simulink model "Step_11"  (R2024b)
settings: Solver=VariableStepAuto  StartTime=0.0  StopTime=100.0  RelTol=1e-3
libraries: simulink x1
settings Model: Creator=Omar

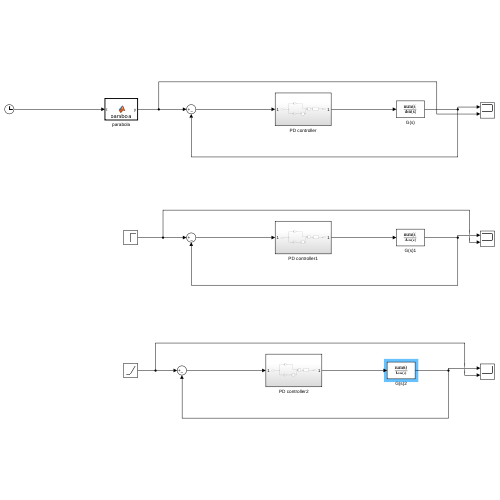
[thumbnail: Simulink's stored preview of the top-level diagram]
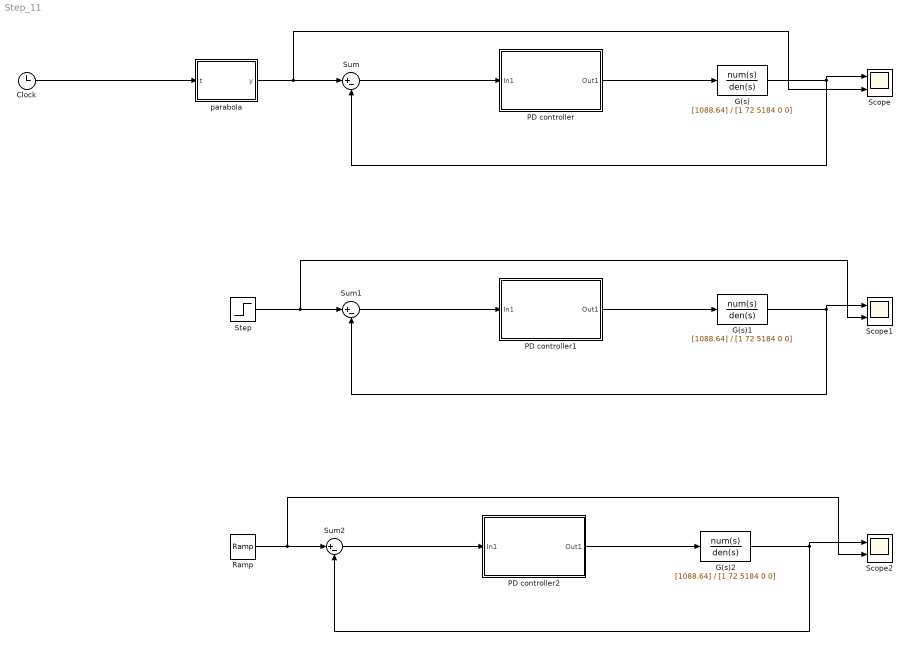
== system Step_11 ==
  Clock : Clock
      settings: Decimation=100
  G(s) : TransferFcn  Numerator=[1088.64]  Denominator=[1 72 5184 0 0]
  G(s)1 : TransferFcn  Numerator=[1088.64]  Denominator=[1 72 5184 0 0]
  G(s)2 : TransferFcn  Numerator=[1088.64]  Denominator=[1 72 5184 0 0]
  PD controller : Subsystem
  PD controller1 : Subsystem
  PD controller2 : Subsystem
  Ramp : simulink/Sources/Ramp  slope=1  start=0  InitialOutput=0
  Scope : Scope  NumInputPorts=2
  Scope1 : Scope  NumInputPorts=2
  Scope2 : Scope  NumInputPorts=2
  Step : Step  SampleTime=0
  Sum : Sum  Inputs=|+-
  Sum1 : Sum  Inputs=|+-
  Sum2 : Sum  Inputs=|+-
  parabola : MATLAB Function  TreatAsAtomicUnit=on
  wires:
  parabola/1(y) -> Scope/2, Sum/1
  G(s)/1 -> Scope/1, Sum/2
  Sum/1 -> PD controller/1(In1)
  PD controller/1(Out1) -> G(s)/1
  G(s)1/1 -> Scope1/1, Sum1/2
  Step/1 -> Scope1/2, Sum1/1
  PD controller1/1(Out1) -> G(s)1/1
  Sum1/1 -> PD controller1/1(In1)
  G(s)2/1 -> Scope2/1, Sum2/2
  Ramp/1 -> Scope2/2, Sum2/1
  PD controller2/1(Out1) -> G(s)2/1
  Sum2/1 -> PD controller2/1(In1)
  Clock/1 -> parabola/1(t)

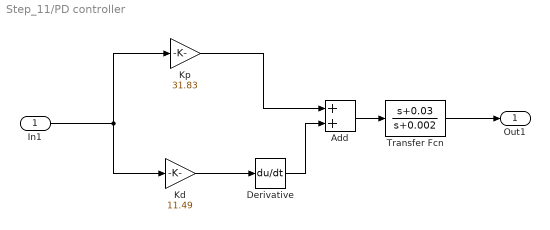
== system Step_11/PD controller ==
  In1 : Inport
  Add : Sum
  Derivative : Derivative
  Kd : Gain  Gain=11.49
  Kp : Gain  Gain=31.83
  Transfer Fcn : TransferFcn  Numerator=[1 0.03]  Denominator=[1 0.002]
  Out1 : Outport
  wires:
  Derivative/1 -> Add/2
  Kp/1 -> Add/1
  In1/1 -> Kp/1, Kd/1
  Kd/1 -> Derivative/1
  Add/1 -> Transfer Fcn/1
  Transfer Fcn/1 -> Out1/1

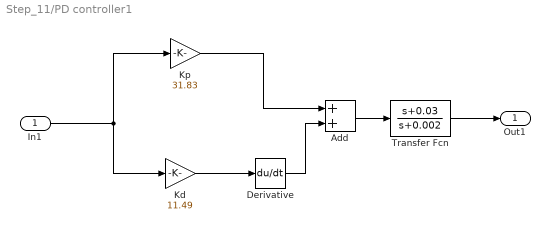
== system Step_11/PD controller1 ==
  In1 : Inport
  Add : Sum
  Derivative : Derivative
  Kd : Gain  Gain=11.49
  Kp : Gain  Gain=31.83
  Transfer Fcn : TransferFcn  Numerator=[1 0.03]  Denominator=[1 0.002]
  Out1 : Outport
  wires:
  Derivative/1 -> Add/2
  Kp/1 -> Add/1
  In1/1 -> Kp/1, Kd/1
  Kd/1 -> Derivative/1
  Add/1 -> Transfer Fcn/1
  Transfer Fcn/1 -> Out1/1

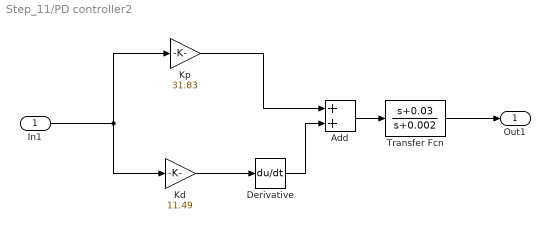
== system Step_11/PD controller2 ==
  In1 : Inport
  Add : Sum
  Derivative : Derivative
  Kd : Gain  Gain=11.49
  Kp : Gain  Gain=31.83
  Transfer Fcn : TransferFcn  Numerator=[1 0.03]  Denominator=[1 0.002]
  Out1 : Outport
  wires:
  Derivative/1 -> Add/2
  Kp/1 -> Add/1
  In1/1 -> Kp/1, Kd/1
  Kd/1 -> Derivative/1
  Add/1 -> Transfer Fcn/1
  Transfer Fcn/1 -> Out1/1

== matlab function Step_11/parabola ==
  data: t input; y output
function y = parabola(t)
    a = 1; % Coefficient for t^2
    b = 0; % Coefficient for t
    c = 0; % Constant term
    y = a * t^2 + b * t + c;
end
